simulink library "foc_blocks"  (R2020b)
settings: Solver=ode45  StartTime=0.0  StopTime=10.0  RelTol=1e-3  EnableMultiTasking=on
values from neighbouring files (symbols this model uses):
  ClockFrequency = 100    [setup_DF_fixp16_alu_av.m]    (also in setup_sim_DF_fixp16_alu.m; setup_verify_DF_fixp16_alu.m)
  constfractionlengthIn = 10    [setup_DF_fixp16_alu_av.m]    (also in setup_sim_DF_fixp16_alu.m; setup_verify_DF_fixp16_alu.m)
  constwordlengthIn = 16    [setup_DF_fixp16_alu_av.m]    (also in setup_sim_DF_fixp16_alu.m; setup_verify_DF_fixp16_alu.m)
  DSPBASampleTime = FoldingFactor / (ClockFrequency * 1e6)    (= 5e-06)    [setup_DF_fixp16_alu_av.m]    (also in setup_sim_DF_fixp16_alu.m; setup_verify_DF_fixp16_alu.m)
  FoldingFactor = 500    [setup_DF_fixp16_alu_av.m]    (also in setup_sim_DF_fixp16_alu.m; setup_verify_DF_fixp16_alu.m)
undefined symbols (not defined in the file or in its folder): AdvDSPBChannelOutDisplay, dpoly, dspba_ChannelInVis, dspba_ChannelOutVis, dspba_internal_get_channel_ports, evalAionMaskParam, latency, primtype, value, x
libraries: DSPBAPrim x559, AlteraGenericMotorLibrary x20, $bdroot x9, DSPBAUtilities x4, DSPBAControl x4
(part 1 of 6)
settings Model: Creator=tchau  LastModifiedBy=shiyaowa
settings DataIOCC: LimitDataPoints=on  SaveFormat=Array  ReturnWorkspaceOutputs=off
settings OptimizationCC: LifeSpan=inf
settings DebuggingCC: SolverPrmCheckMsg=warning  SFUnexpectedBacktrackingDiag=warning  SFNoUnconditionalDefaultTransitionDiag=warning  SFExecutionAtInitializationDiag=none  ArithmeticOperatorsInVariantConditions=warning
settings HardwareCC: ProdBitPerPointer=32  ProdBitPerSizeT=32  ProdBitPerPtrDiffT=32  ProdLargestAtomicFloat=None  ProdIntDivRoundTo=Undefined  ProdEndianess=Unspecified  ProdWordSize=32  ProdHWDeviceType=32-bit Generic
settings ModelReferenceCC: PropagateSignalLabelsOutOfModel=off
settings SFSimCC: SimUseLocalCustomCode=off  CustomCodeUndefinedFunction=UseInterfaceOnly
settings RTWCC: RTWUseLocalCustomCode=off
settings CodeAppCC: StateflowObjectComments=on
settings GRTTargetCC: TargetLangStandard=C89/C90 (ANSI)
settings ConfigComp: CovMetricSettings=dw  CovSaveCumulativeToWorkspaceVar=on  CovSaveSingleToWorkspaceVar=on  CovExternalEMLEnable=off

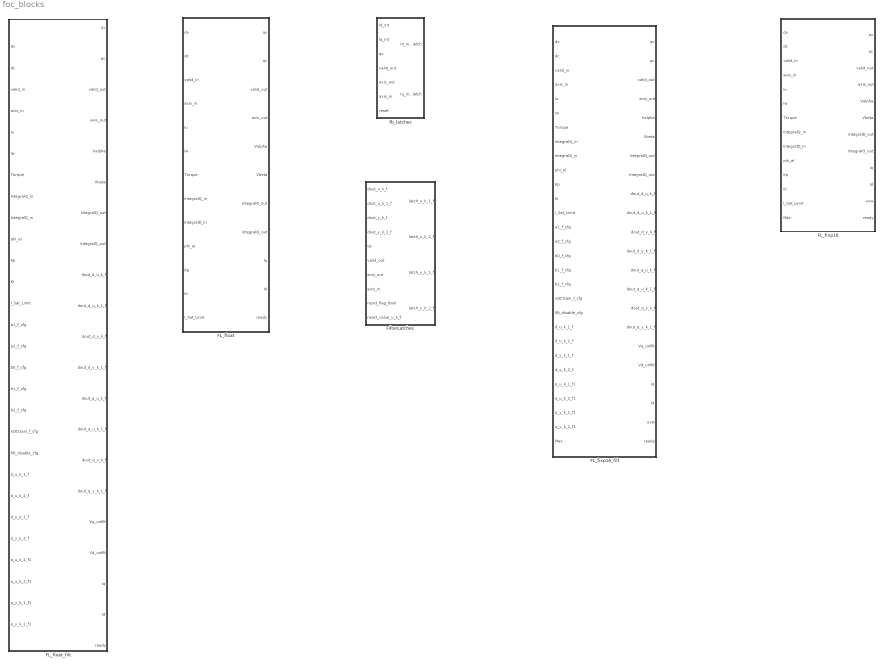
== system foc_blocks ==
  FL_fixp16 : Subsystem
  FL_fixp16_filt : Subsystem
  FL_float : Subsystem
  FL_float_filt : Subsystem
  FilterLatches : Subsystem
  fb_latches : Subsystem

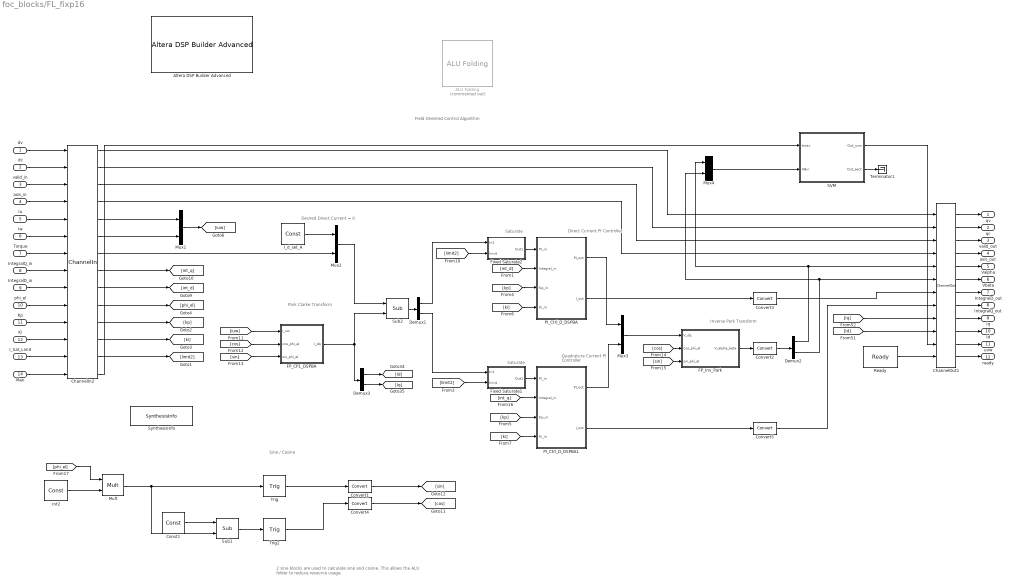
== system foc_blocks/FL_fixp16 ==
  note: Field Oriented Control Algorithm
  note: Sine / Cosine
  note: Saturate
  note: Saturate
  note: Park Clarke
      |  Transform
  note: Inverse Park
      |  Transform
  note: Desired Direct Current = 0
  note: Direct Current
      | PI Controller
  note: Quadrature Current
      | PI Controller
  note: 2 sine blocks are used to calculate sine and cosine.
      | This allows the ALU folder to reduce resource usage.
  dv : Inport
  dc : Inport  Port=2
  valid_in : Inport  Port=3
  axis_in : Inport  Port=4
  Iu : Inport  Port=5
  Iw : Inport  Port=6
  Torque : Inport  Port=7
  IntegralQ_in : Inport  Port=8
  IntegralD_in : Inport  Port=9
  phi_el : Inport  Port=10
  Kp : Inport  Port=11
  Ki : Inport  Port=12
  I_Sat_Limit : Inport  Port=13
  Max : Inport  Port=14
  ALU Folding : DSPBAUtilities/ALU Folding  Description=Enables the new folder. When this block is placed in a subsystem, all primitive subsystems at the level it is placed and below will be passed to the folder. DSP Builder will then generate folded subsystems which can be placed back into the existing design.  Commented=on  version=20130913  genModelFileName=folded_model.xml  sampleRate=SampleRate  numChannels=1  maxLatency=LatencyConstraint  inputFormat=Parallel  outputFormat=Parallel  latchOutputs=off  originalRate=off  hasIdleState=off  padInputs=off  simRate=Data rate
  Altera DSP Builder Advanced : AlteraGenericMotorLibrary/FP_Cur_Ctrl_DSPBA/Altera DSP Builder Advanced  SystemSampleTime=-1  VariantActivationTime=update diagram  Latency=0  AutoFrameSizeCalculation=off
  ChannelIn2 : DSPBAPrim/ChannelIn  primtype=channelin  nInputs=dspba_internal_get_channel_ports(gcb)  nOutputs=dspba_internal_get_channel_ports(gcb)  omode=Inherit via internal rule  otype=sfix(16)  scale=2^-15  rndmethod=Unbiased  factor=1  satmethod=Symmetric  shift_vec=[0 1 2 -1]  value=12  inPortNames=['v'; 'c'; '0'; '1'; '2'; '3'; '4'; '5'; '6'; '7'; '8'; '9'; 'A'; 'B'; 'D'; 'E'; 'F'; 'G'; 'H'; 'I'; 'J'; 'K'; 'L'; 'M'; 'N'; 'O'; 'P'; 'Q'; 'R'; 'S'; 'T'; 'U'; 'W'; 'X'; 'Y'; 'Z']  outPortNames=['v'; 'c'; '0'; '1'; '2'; '3'; '4'; '5'; '6'; '7'; '8'; '9'; 'A'; 'B'; 'D'; 'E'; 'F'; 'G'; 'H'; 'I'; 'J'; 'K'; 'L'; 'M'; 'N'; 'O'; 'P'; 'Q'; 'R'; 'S'; 'T'; 'U'; 'W'; 'X'; 'Y'; 'Z']  dspbaimage=dspba_prim.jpg  text=fprintf('In');  style=Optimised  dataSignals=12  foldingEnabled=off  channels=1  sampleRate=200  packetBeginPresent=off  packetBeginEnabled=off  visibilities=dspba_ChannelInVis(gcb)  latencyCorrection=0  scheduleOrigin=off  version=20141013
  ChannelOut1 : DSPBAPrim/ChannelOut  primtype=channelout  nInputs=dspba_internal_get_channel_ports(gcb)  nOutputs=dspba_internal_get_channel_ports(gcb)  omode=Inherit via internal rule  otype=sfix(16)  scale=2^-15  rndmethod=Unbiased  factor=1  satmethod=Symmetric  shift_vec=[0 1 2 -1]  value=10  inPortNames=['v'; 'c'; '0'; '1'; '2'; '3'; '4'; '5'; '6'; '7'; '8'; '9'; 'A'; 'B'; 'D'; 'E'; 'F'; 'G'; 'H'; 'I'; 'J'; 'K'; 'L'; 'M'; 'N'; 'O'; 'P'; 'Q'; 'R'; 'S'; 'T'; 'U'; 'W'; 'X'; 'Y'; 'Z']  outPortNames=['v'; 'c'; '0'; '1'; '2'; '3'; '4'; '5'; '6'; '7'; '8'; '9'; 'A'; 'B'; 'D'; 'E'; 'F'; 'G'; 'H'; 'I'; 'J'; 'K'; 'L'; 'M'; 'N'; 'O'; 'P'; 'Q'; 'R'; 'S'; 'T'; 'U'; 'W'; 'X'; 'Y'; 'Z']  dspbaimage=dspba_prim.jpg  text=fprintf('Out%s', AdvDSPBChannelOutDisplay(latency));  style=Optimised  dataSignals=10  foldingEnabled=off  channels=1  sampleRate=200  packetBeginPresent=off  packetBeginEnabled=off  visibilities=dspba_ChannelOutVis(gcb)  latency=22  latencyCorrection=0  version=20141013
  Const1 : DSPBAPrim/Const  primtype=const  nInputs=0  nOutputs=1  omode=Specify via dialog  otype=constOTypeIn  scale=constScaleIn  rndmethod=Unbiased  factor=1  satmethod=Symmetric  shift_vec=[0 1 2 -1]  value=1/2  inPortNames=['+'; '+';]  outPortNames=[' ']  dspbaimage=dspba_prim.jpg  text=fprintf('%s', num2str(value));  style=Optimised  visibilities=8 + 1024  floatPrecision=float26_m17  version=20120820
  Convert{1,3..5} (4 alike) : DSPBAPrim/Convert  primtype=convert  nInputs=1  nOutputs=1  omode=Specify via dialog  otype=constOTypeIn  scale=constScaleIn  rndmethod=Truncate  factor=1  satmethod=None  shift_vec=[0 1 2 -1]  value=round([0:255]/17)  inPortNames=[' '; ' ';]  outPortNames=[' '; 'c']  dspbaimage=dspba_prim.jpg  text=fprintf('convert');  style=Optimised  visibilities=8+64+256  clipdetect=off  floatPrecision=float32_m23  advOptions=[]  version=20130211
  Convert2 : DSPBAPrim/Convert  primtype=convert  nInputs=1  nOutputs=1  omode=Specify via dialog  otype=constOType  scale=constScale  rndmethod=Truncate  factor=1  satmethod=None  shift_vec=[0 1 2 -1]  value=round([0:255]/17)  inPortNames=[' '; ' ';]  outPortNames=[' '; 'c']  dspbaimage=dspba_prim.jpg  text=fprintf('convert');  style=Optimised  visibilities=8+64+256  clipdetect=off  floatPrecision=float32_m23  advOptions=[]  version=20130211
  Demux1 : Demux  Outputs=2
  Demux2 : Demux  Outputs=2
  Demux3 : Demux  Outputs=2
  FP_CP1_DSPBA : Subsystem  Description=Clarke & Park Transforms
      mask Display: color('white');port_label('output', 1, 'I_dq'); port_label('input', 1, 'I_uw');port_label('input', 2, 'cos_phi');port_label('input', 3, 'sin_phi');
  FP_Inv_Park : Subsystem  Description=Inverse Park & Clarke transforms
      mask Display: color('white');port_label('output', 1, 'V_alpha_beta'); port_label('input', 1, 'V_dq');port_label('input', 2, 'cos_phi');port_label('input', 3, 'sin_phi');
  Fixed Saturate1 : Subsystem
  Fixed Saturate2 : Subsystem
  I_d_set_A : DSPBAPrim/Const  primtype=const  nInputs=0  nOutputs=1  omode=Specify via dialog  otype=constOTypeIn  scale=constScaleIn  rndmethod=Unbiased  factor=1  satmethod=Symmetric  shift_vec=[0 1 2 -1]  value=0  inPortNames=['+'; '+';]  outPortNames=[' ']  dspbaimage=dspba_prim.jpg  text=fprintf('%s', num2str(value));  style=Optimised  visibilities=8 + 1024  floatPrecision=float32_m23  version=20120820
  Mult : DSPBAPrim/Mult  primtype=mult  nInputs=2  nOutputs=1  omode=Specify via dialog  otype=constOTypeIn  scale=constScaleIn  rndmethod=Unbiased  factor=1  satmethod=Symmetric  shift_vec=[0 1 2 -1]  value=0  inPortNames=[' '; ' ';]  outPortNames=[' ']  dspbaimage=dspba_prim.jpg  text=fprintf('X');  style=Optimised  visibilities=8  floatPrecision=float32_m23  floatRounding=correct  advOptions=[]  version=20130115
  Mux{1..4} (4 alike) : Mux  Inputs=2
  PI_Ctrl_D_DSPBA : Subsystem
  PI_Ctrl_D_DSPBA1 : Subsystem
  Ready : DSPBAPrim/Ready  primtype=ready  nInputs=0  nOutputs=1  omode=Inherit via internal rule  otype=ufix(1)  scale=2^-0  rndmethod=Unbiased  factor=1  satmethod=Asymmetric  shift_vec=[]  value=1  inPortNames=['']  outPortNames=[' ']  dspbaimage=dspba_prim.jpg  text=fprintf('Ready');  style=Processor  visibilities=0  floatPrecision=float32_m23  version=20131024
  SVM : Subsystem
  Sub1 : DSPBAPrim/Sub  primtype=sub  nInputs=2  nOutputs=1  omode=Inherit via internal rule  otype=sfix(16)  scale=2^-15  rndmethod=Unbiased  factor=1  satmethod=Symmetric  shift_vec=[0 1 2 -1]  value=0  inPortNames=['+'; '-';]  outPortNames=[' ']  dspbaimage=dspba_prim.jpg  text=fprintf('-');  style=Optimised  visibilities=8  floatRounding=correct  advOptions=[]  version=20130115
  Sub2 : DSPBAPrim/Sub  primtype=sub  nInputs=2  nOutputs=1  omode=Inherit via internal rule  otype=sfix(16)  scale=2^-15  rndmethod=Unbiased  factor=1  satmethod=Symmetric  shift_vec=[0 1 2 -1]  value=0  inPortNames=['+'; '-';]  outPortNames=[' ']  dspbaimage=dspba_prim.jpg  text=fprintf('-');  style=Optimised  visibilities=8  floatRounding=correct  advOptions=[]  version=20130115
  SynthesisInfo : DSPBAPrim/SynthesisInfo  primtype=synthinfo  nInputs=0  nOutputs=0  omode=Inherit via internal rule  otype=sfix(16)  scale=2^-15  rndmethod=Truncate  factor=1  satmethod=Symmetric  shift_vec=[0 1 2 -1]  value=99  inPortNames=[' '; ' ';]  outPortNames=[' ']  dspbaimage=dspba_prim_ctrl.jpg  text=fprintf('Style=%s', style);  style=Scheduled  visibilities=32768  constraintInUse=off  constraintRelation=>  constraintLimit=2  bitAccurate=off  version=20150220
  Terminator1 : Terminator
  Trig : DSPBAPrim/Trig  primtype=trigfunc  nInputs=1  nOutputs=1  omode=Inherit via internal rule  otype=sfix(16)  scale=2^-15  rndmethod=Unbiased  factor=1  satmethod=Symmetric  shift_vec=[0 1 2 -1]  value=round([0:255]/17)  inPortNames=[' '; ' ';]  outPortNames=[' ']  dspbaimage=dspba_prim_float.jpg  text=fprintf('sin(a)');  style=Optimised  visibilities=2^17+2^18  functionExpr=sin(pi*x)  advOptions=[]  version=20140803
  Trig2 : DSPBAPrim/Trig  primtype=trigfunc  nInputs=1  nOutputs=1  omode=Inherit via internal rule  otype=sfix(16)  scale=2^-15  rndmethod=Unbiased  factor=1  satmethod=Symmetric  shift_vec=[0 1 2 -1]  value=round([0:255]/17)  inPortNames=[' '; ' ';]  outPortNames=[' ']  dspbaimage=dspba_prim_float.jpg  text=fprintf('sin(a)');  style=Optimised  visibilities=2^17+2^18  functionExpr=sin(pi*x)  advOptions=[]  version=20140803
  cst2 : DSPBAPrim/Const  primtype=const  nInputs=0  nOutputs=1  omode=Specify via dialog  otype=constOTypeIn  scale=constScaleIn  rndmethod=Unbiased  factor=1  satmethod=Symmetric  shift_vec=[0 1 2 -1]  value=2  inPortNames=['+'; '+';]  outPortNames=[' ']  dspbaimage=dspba_prim.jpg  text=fprintf('%s', num2str(value));  style=Optimised  visibilities=8 + 1024  floatPrecision=float26_m17  version=20120820
  qv : Outport
  qc : Outport  Port=2
  valid_out : Outport  Port=3
  axis_out : Outport  Port=4
  Valpha : Outport  Port=5
  Vbeta : Outport  Port=6
  IntegralD_out : Outport  Port=7
  IntegralQ_out : Outport  Port=8
  Iq : Outport  Port=9
  Id : Outport  Port=10
  uvw : Outport  Port=11
  ready : Outport  Port=12
  wires:
  SVM/2(Out_sect) -> Terminator1/1
  Ready/1 -> ChannelOut1/12
  ChannelOut1/12 -> ready/1
  SVM/1(Out_uvw) -> ChannelOut1/11
  ChannelOut1/11 -> uvw/1
  ChannelIn2/14 -> SVM/1(tmax)
  Max/1 -> ChannelIn2/14
  Mux4/1 -> SVM/2(ABin)
  Mux2/1 -> Sub2/1
  ChannelIn2/12 -> [ki]
  ChannelIn2/11 -> [kp]
  ChannelIn2/10 -> [phi_el]
  ChannelIn2/9 -> [int_d]
  ChannelIn2/8 -> [int_q]
  ChannelIn2/7 -> Mux2/2
  ChannelIn2/6 -> Mux1/2
  ChannelIn2/5 -> Mux1/1
  Sub1/1 -> Trig2/1
  Mult/1 -> Sub1/2, Trig/1
  Const1/1 -> Sub1/1
  Convert4/1 -> [cos]
  Convert1/1 -> [sin]
  Trig2/1 -> Convert4/1
  Trig/1 -> Convert1/1
  cst2/1 -> Mult/2
  [phi_el] -> Mult/1
  ChannelIn2/4 -> ChannelOut1/4
  [sin] -> FP_Inv_Park/3(sin_phi_el)
  [cos] -> FP_Inv_Park/2(cos_phi_el)
  Convert2/1 -> Demux2/1
  Mux1/1 -> [iuw]
  [sin] -> FP_CP1_DSPBA/3(sin_phi_el)
  [cos] -> FP_CP1_DSPBA/2(cos_phi_el)
  [iuw] -> FP_CP1_DSPBA/1(I_uw)
  [limit2] -> Fixed Saturate2/2(limit)
  [ki] -> PI_Ctrl_D_DSPBA/4(Ki_in)
  [kp] -> PI_Ctrl_D_DSPBA/3(Kp_in)
  [int_d] -> PI_Ctrl_D_DSPBA/2(Integral_in)
  [limit2] -> Fixed Saturate1/2(limit)
  [ki] -> PI_Ctrl_D_DSPBA1/4(Ki_in)
  [kp] -> PI_Ctrl_D_DSPBA1/3(Kp_in)
  [int_q] -> PI_Ctrl_D_DSPBA1/2(Integral_in)
  Demux1/2 -> Fixed Saturate1/1(In1)
  Demux1/1 -> Fixed Saturate2/1(In1)
  Sub2/1 -> Demux1/1
  I_d_set_A/1 -> Mux2/1
  Demux2/2 -> ChannelOut1/6, Mux4/2
  Demux2/1 -> ChannelOut1/5, Mux4/1
  FP_Inv_Park/1(V_alpha_beta) -> Convert2/1
  Mux3/1 -> FP_Inv_Park/1(V_dq)
  PI_Ctrl_D_DSPBA1/1(PI_out) -> Mux3/2
  PI_Ctrl_D_DSPBA/1(PI_out) -> Mux3/1
  Convert3/1 -> ChannelOut1/7
  PI_Ctrl_D_DSPBA/2(I_out) -> Convert3/1
  Convert5/1 -> ChannelOut1/8
  PI_Ctrl_D_DSPBA1/2(I_out) -> Convert5/1
  Fixed Saturate2/1(Out1) -> PI_Ctrl_D_DSPBA/1(PI_in)
  Fixed Saturate1/1(Out1) -> PI_Ctrl_D_DSPBA1/1(PI_in)
  ChannelIn2/3 -> ChannelOut1/3
  ChannelIn2/2 -> ChannelOut1/2
  ChannelIn2/1 -> ChannelOut1/1
  dv/1 -> ChannelIn2/1
  dc/1 -> ChannelIn2/2
  valid_in/1 -> ChannelIn2/3
  axis_in/1 -> ChannelIn2/4
  Iu/1 -> ChannelIn2/5
  Iw/1 -> ChannelIn2/6
  Torque/1 -> ChannelIn2/7
  IntegralQ_in/1 -> ChannelIn2/8
  IntegralD_in/1 -> ChannelIn2/9
  phi_el/1 -> ChannelIn2/10
  Kp/1 -> ChannelIn2/11
  Ki/1 -> ChannelIn2/12
  ChannelOut1/1 -> qv/1
  ChannelOut1/2 -> qc/1
  ChannelOut1/3 -> valid_out/1
  ChannelOut1/4 -> axis_out/1
  ChannelOut1/5 -> Valpha/1
  ChannelOut1/6 -> Vbeta/1
  ChannelOut1/7 -> IntegralD_out/1
  ChannelOut1/8 -> IntegralQ_out/1
  FP_CP1_DSPBA/1(I_dq) -> Sub2/2, Demux3/1
  Demux3/1 -> [Id]
  Demux3/2 -> [Iq]
  [Iq] -> ChannelOut1/9
  [Id] -> ChannelOut1/10
  ChannelOut1/9 -> Iq/1
  ChannelOut1/10 -> Id/1
  I_Sat_Limit/1 -> ChannelIn2/13
  ChannelIn2/13 -> [limit2]

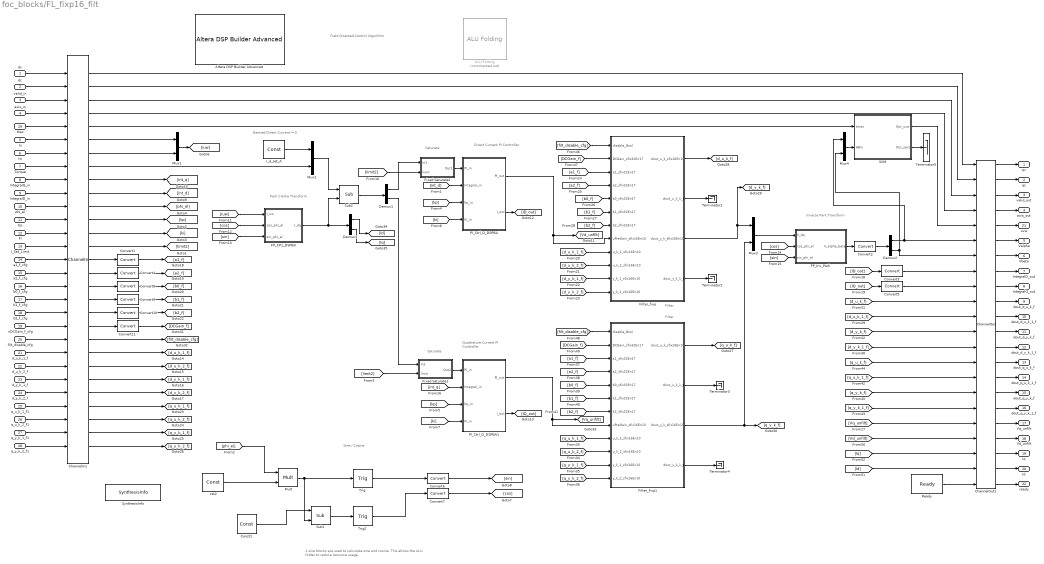
== system foc_blocks/FL_fixp16_filt ==
  note: Sine / Cosine
  note: Filter
  note: Filter
  note: Field Oriented Control Algorithm
  note: Saturate
  note: Saturate
  note: Park Clarke
      |  Transform
  note: Inverse Park
      |  Transform
  note: Desired Direct Current = 0
  note: Direct Current
      | PI Controller
  note: Quadrature Current
      | PI Controller
  note: 2 sine blocks are used to calculate sine and cosine.
      | This allows the ALU folder to reduce resource usage.
  dv : Inport
  dc : Inport  Port=2
  valid_in : Inport  Port=3
  axis_in : Inport  Port=4
  Iu : Inport  Port=5
  Iw : Inport  Port=6
  Torque : Inport  Port=7
  IntegralQ_in : Inport  Port=8
  IntegralD_in : Inport  Port=9
  phi_el : Inport  Port=10
  Kp : Inport  Port=11
  Ki : Inport  Port=12
  I_Sat_Limit : Inport  Port=13
  a1_f_cfg : Inport  Port=14
  a2_f_cfg : Inport  Port=15
  b0_f_cfg : Inport  Port=16
  b1_f_cfg : Inport  Port=17
  b2_f_cfg : Inport  Port=18
  xDCGain_f_cfg : Inport  Port=19
  filt_disable_cfg : Inport  Port=20
  d_u_k_1_f : Inport  Port=21
  d_u_k_2_f : Inport  Port=22
  d_y_k_1_f : Inport  Port=23
  d_y_k_2_f : Inport  Port=24
  q_u_k_1_f1 : Inport  Port=25
  q_u_k_2_f1 : Inport  Port=26
  q_y_k_1_f1 : Inport  Port=27
  q_y_k_2_f1 : Inport  Port=28
  Max : Inport  Port=29
  ALU Folding : DSPBAUtilities/ALU Folding  Description=Enables the new folder. When this block is placed in a subsystem, all primitive subsystems at the level it is placed and below will be passed to the folder. DSP Builder will then generate folded subsystems which can be placed back into the existing design.  Commented=on  version=20130913  genModelFileName=folded_model.xml  sampleRate=SampleRate  numChannels=1  maxLatency=LatencyConstraint  inputFormat=Parallel  outputFormat=Parallel  latchOutputs=off  originalRate=off  hasIdleState=off  padInputs=off  simRate=Data rate
  Altera DSP Builder Advanced : AlteraGenericMotorLibrary/FP_Cur_Ctrl_DSPBA/Altera DSP Builder Advanced  SystemSampleTime=-1  VariantActivationTime=update diagram  Latency=0  AutoFrameSizeCalculation=off
  ChannelIn1 : DSPBAPrim/ChannelIn  primtype=channelin  nInputs=dspba_internal_get_channel_ports(gcb)  nOutputs=dspba_internal_get_channel_ports(gcb)  omode=Inherit via internal rule  otype=sfix(16)  scale=2^-15  rndmethod=Unbiased  factor=1  satmethod=Symmetric  shift_vec=[0 1 2 -1]  value=27  inPortNames=['v'; 'c'; '0'; '1'; '2'; '3'; '4'; '5'; '6'; '7'; '8'; '9'; 'A'; 'B'; 'D'; 'E'; 'F'; 'G'; 'H'; 'I'; 'J'; 'K'; 'L'; 'M'; 'N'; 'O'; 'P'; 'Q'; 'R'; 'S'; 'T'; 'U'; 'W'; 'X'; 'Y'; 'Z']  outPortNames=['v'; 'c'; '0'; '1'; '2'; '3'; '4'; '5'; '6'; '7'; '8'; '9'; 'A'; 'B'; 'D'; 'E'; 'F'; 'G'; 'H'; 'I'; 'J'; 'K'; 'L'; 'M'; 'N'; 'O'; 'P'; 'Q'; 'R'; 'S'; 'T'; 'U'; 'W'; 'X'; 'Y'; 'Z']  dspbaimage=dspba_prim.jpg  text=fprintf('In');  style=Optimised  dataSignals=27  foldingEnabled=off  channels=1  sampleRate=ClockFrequency/FoldingFactor  packetBeginPresent=off  packetBeginEnabled=off  visibilities=dspba_ChannelInVis(gcb)  latencyCorrection=0  scheduleOrigin=off  version=20141013
  ChannelOut1 : DSPBAPrim/ChannelOut  primtype=channelout  nInputs=dspba_internal_get_channel_ports(gcb)  nOutputs=dspba_internal_get_channel_ports(gcb)  omode=Inherit via internal rule  otype=sfix(16)  scale=2^-15  rndmethod=Unbiased  factor=1  satmethod=Symmetric  shift_vec=[0 1 2 -1]  value=20  inPortNames=['v'; 'c'; '0'; '1'; '2'; '3'; '4'; '5'; '6'; '7'; '8'; '9'; 'A'; 'B'; 'D'; 'E'; 'F'; 'G'; 'H'; 'I'; 'J'; 'K'; 'L'; 'M'; 'N'; 'O'; 'P'; 'Q'; 'R'; 'S'; 'T'; 'U'; 'W'; 'X'; 'Y'; 'Z']  outPortNames=['v'; 'c'; '0'; '1'; '2'; '3'; '4'; '5'; '6'; '7'; '8'; '9'; 'A'; 'B'; 'D'; 'E'; 'F'; 'G'; 'H'; 'I'; 'J'; 'K'; 'L'; 'M'; 'N'; 'O'; 'P'; 'Q'; 'R'; 'S'; 'T'; 'U'; 'W'; 'X'; 'Y'; 'Z']  dspbaimage=dspba_prim.jpg  text=fprintf('Out%s', AdvDSPBChannelOutDisplay(latency));  style=Optimised  dataSignals=20  foldingEnabled=off  channels=1  sampleRate=ClockFrequency/FoldingFactor  packetBeginPresent=off  packetBeginEnabled=off  visibilities=dspba_ChannelOutVis(gcb)  latency=17  latencyCorrection=0  version=20141013
  Const1 : DSPBAPrim/Const  primtype=const  nInputs=0  nOutputs=1  omode=Specify via dialog  otype=constOTypeIn  scale=constScaleIn  rndmethod=Unbiased  factor=1  satmethod=Symmetric  shift_vec=[0 1 2 -1]  value=1/2  inPortNames=['+'; '+';]  outPortNames=[' ']  dspbaimage=dspba_prim.jpg  text=fprintf('%s', num2str(value));  style=Optimised  visibilities=8 + 1024  floatPrecision=float26_m17  version=20120820
  Convert{1,3..11} (10 alike) : DSPBAPrim/Convert  primtype=convert  nInputs=1  nOutputs=1  omode=Specify via dialog  otype=constOTypeIn  scale=constScaleIn  rndmethod=Truncate  factor=1  satmethod=None  shift_vec=[0 1 2 -1]  value=round([0:255]/17)  inPortNames=[' '; ' ';]  outPortNames=[' '; 'c']  dspbaimage=dspba_prim.jpg  text=fprintf('convert');  style=Optimised  visibilities=8+64+256  clipdetect=off  floatPrecision=float32_m23  advOptions=[]  version=20130211
  Convert2 : DSPBAPrim/Convert  primtype=convert  nInputs=1  nOutputs=1  omode=Specify via dialog  otype=constOType  scale=constScale  rndmethod=Truncate  factor=1  satmethod=None  shift_vec=[0 1 2 -1]  value=round([0:255]/17)  inPortNames=[' '; ' ';]  outPortNames=[' '; 'c']  dspbaimage=dspba_prim.jpg  text=fprintf('convert');  style=Optimised  visibilities=8+64+256  clipdetect=off  floatPrecision=float32_m23  advOptions=[]  version=20130211
  Demux1 : Demux  Outputs=2
  Demux2 : Demux  Outputs=2
  Demux3 : Demux  Outputs=2
  FP_CP1_DSPBA : Subsystem  Description=Clarke & Park Transforms
      mask Display: color('white');port_label('output', 1, 'I_dq'); port_label('input', 1, 'I_uw');port_label('input', 2, 'cos_phi');port_label('input', 3, 'sin_phi');
  FP_Inv_Park : Subsystem  Description=Inverse Park & Clarke transforms
      mask Display: color('white');port_label('output', 1, 'V_alpha_beta'); port_label('input', 1, 'V_dq');port_label('input', 2, 'cos_phi');port_label('input', 3, 'sin_phi');
  Filter_fixp : Subsystem
  Filter_fixp1 : Subsystem
  Fixed Saturate1 : Subsystem
  Fixed Saturate2 : Subsystem
  I_d_set_A : DSPBAPrim/Const  primtype=const  nInputs=0  nOutputs=1  omode=Specify via dialog  otype=constOTypeIn  scale=constScaleIn  rndmethod=Unbiased  factor=1  satmethod=Symmetric  shift_vec=[0 1 2 -1]  value=0  inPortNames=['+'; '+';]  outPortNames=[' ']  dspbaimage=dspba_prim.jpg  text=fprintf('%s', num2str(value));  style=Optimised  visibilities=8 + 1024  floatPrecision=float32_m23  version=20120820
  Mult : DSPBAPrim/Mult  primtype=mult  nInputs=2  nOutputs=1  omode=Specify via dialog  otype=constOTypeIn  scale=constScaleIn  rndmethod=Unbiased  factor=1  satmethod=Symmetric  shift_vec=[0 1 2 -1]  value=0  inPortNames=[' '; ' ';]  outPortNames=[' ']  dspbaimage=dspba_prim.jpg  text=fprintf('X');  style=Optimised  visibilities=8  floatPrecision=float32_m23  floatRounding=correct  advOptions=[]  version=20130115
  Mux{1..4} (4 alike) : Mux  Inputs=2
  PI_Ctrl_D_DSPBA : Subsystem
  PI_Ctrl_D_DSPBA1 : Subsystem
  Ready : DSPBAPrim/Ready  primtype=ready  nInputs=0  nOutputs=1  omode=Inherit via internal rule  otype=ufix(1)  scale=2^-0  rndmethod=Unbiased  factor=1  satmethod=Asymmetric  shift_vec=[]  value=1  inPortNames=['']  outPortNames=[' ']  dspbaimage=dspba_prim.jpg  text=fprintf('Ready');  style=Processor  visibilities=0  floatPrecision=float32_m23  version=20131024
  SVM : Subsystem
  Sub1 : DSPBAPrim/Sub  primtype=sub  nInputs=2  nOutputs=1  omode=Inherit via internal rule  otype=sfix(16)  scale=2^-15  rndmethod=Unbiased  factor=1  satmethod=Symmetric  shift_vec=[0 1 2 -1]  value=0  inPortNames=['+'; '-';]  outPortNames=[' ']  dspbaimage=dspba_prim.jpg  text=fprintf('-');  style=Optimised  visibilities=8  floatRounding=correct  advOptions=[]  version=20130115
  Sub2 : DSPBAPrim/Sub  primtype=sub  nInputs=2  nOutputs=1  omode=Inherit via internal rule  otype=sfix(16)  scale=2^-15  rndmethod=Unbiased  factor=1  satmethod=Symmetric  shift_vec=[0 1 2 -1]  value=0  inPortNames=['+'; '-';]  outPortNames=[' ']  dspbaimage=dspba_prim.jpg  text=fprintf('-');  style=Optimised  visibilities=8  floatRounding=correct  advOptions=[]  version=20130115
  SynthesisInfo : DSPBAPrim/SynthesisInfo  primtype=synthinfo  nInputs=0  nOutputs=0  omode=Inherit via internal rule  otype=sfix(16)  scale=2^-15  rndmethod=Truncate  factor=1  satmethod=Symmetric  shift_vec=[0 1 2 -1]  value=99  inPortNames=[' '; ' ';]  outPortNames=[' ']  dspbaimage=dspba_prim_ctrl.jpg  text=fprintf('Style=%s', style);  style=Scheduled  visibilities=32768  constraintInUse=off  constraintRelation=>  constraintLimit=2  bitAccurate=off  version=20150220
  Terminator{1..5} (5 alike) : Terminator
  Trig : DSPBAPrim/Trig  primtype=trigfunc  nInputs=1  nOutputs=1  omode=Inherit via internal rule  otype=sfix(16)  scale=2^-15  rndmethod=Unbiased  factor=1  satmethod=Symmetric  shift_vec=[0 1 2 -1]  value=round([0:255]/17)  inPortNames=[' '; ' ';]  outPortNames=[' ']  dspbaimage=dspba_prim_float.jpg  text=fprintf('sin(a)');  style=Optimised  visibilities=2^17+2^18  functionExpr=sin(pi*x)  advOptions=[]  version=20140803
  Trig2 : DSPBAPrim/Trig  primtype=trigfunc  nInputs=1  nOutputs=1  omode=Inherit via internal rule  otype=sfix(16)  scale=2^-15  rndmethod=Unbiased  factor=1  satmethod=Symmetric  shift_vec=[0 1 2 -1]  value=round([0:255]/17)  inPortNames=[' '; ' ';]  outPortNames=[' ']  dspbaimage=dspba_prim_float.jpg  text=fprintf('sin(a)');  style=Optimised  visibilities=2^17+2^18  functionExpr=sin(pi*x)  advOptions=[]  version=20140803
  cst2 : DSPBAPrim/Const  primtype=const  nInputs=0  nOutputs=1  omode=Specify via dialog  otype=constOTypeIn  scale=constScaleIn  rndmethod=Unbiased  factor=1  satmethod=Symmetric  shift_vec=[0 1 2 -1]  value=2  inPortNames=['+'; '+';]  outPortNames=[' ']  dspbaimage=dspba_prim.jpg  text=fprintf('%s', num2str(value));  style=Optimised  visibilities=8 + 1024  floatPrecision=float26_m17  version=20120820
  qv : Outport
  qc : Outport  Port=2
  valid_out : Outport  Port=3
  axis_out : Outport  Port=4
  Valpha : Outport  Port=5
  Vbeta : Outport  Port=6
  IntegralD_out : Outport  Port=7
  IntegralQ_out : Outport  Port=8
  dout_d_u_k_f : Outport  Port=9
  dout_d_u_k_1_f : Outport  Port=10
  dout_d_y_k_f : Outport  Port=11
  dout_d_y_k_1_f : Outport  Port=12
  dout_q_u_k_f : Outport  Port=13
  dout_q_u_k_1_f : Outport  Port=14
  dout_q_y_k_f : Outport  Port=15
  dout_q_y_k_1_f : Outport  Port=16
  Vq_unfilt : Outport  Port=17
  Vd_unfilt : Outport  Port=18
  Iq : Outport  Port=19
  Id : Outport  Port=20
  uvw : Outport  Port=21
  ready : Outport  Port=22
  wires:
  Sub1/1 -> Trig2/1
  Mult/1 -> Sub1/2, Trig/1
  Const1/1 -> Sub1/1
  Convert7/1 -> [cos]
  Convert6/1 -> [sin]
  Trig2/1 -> Convert7/1
  Trig/1 -> Convert6/1
  cst2/1 -> Mult/2
  [phi_el] -> Mult/1
  PI_Ctrl_D_DSPBA1/1(PI_out) -> Filter_fixp1/8(uPreGain_sfix16En10), [Vq_unfilt]
  PI_Ctrl_D_DSPBA/1(PI_out) -> [Vd_unfilt], Filter_fixp/8(uPreGain_sfix16En10)
  Demux3/2 -> [Iq]
  Demux3/1 -> [Id]
  [DCGain_f] -> Filter_fixp1/2(DCGain_sfix32En17)
  [filt_disable_cfg] -> Filter_fixp1/1(disable_Bool)
  Filter_fixp1/1(dout_u_k_sfix16En10) -> [q_u_k_f]
  Filter_fixp1/2(dout_u_k_1_f) -> Terminator3/1
  Filter_fixp1/4(dout_y_k_1_f) -> Terminator4/1
  [a1_f] -> Filter_fixp1/3(a1_sfix32En17)
  [a2_f] -> Filter_fixp1/4(a2_sfix32En17)
  [b0_f] -> Filter_fixp1/5(b0_sfix32En17)
  [b1_f] -> Filter_fixp1/6(b1_sfix32En17)
  [b2_f] -> Filter_fixp1/7(b2_sfix32En17)
  [q_y_k_2_f] -> Filter_fixp1/12(y_k_2_sfix16En10)
  [q_y_k_1_f] -> Filter_fixp1/11(y_k_1_sfix16En10)
  [q_u_k_2_f] -> Filter_fixp1/10(u_k_2_sfix16En10)
  [q_u_k_1_f] -> Filter_fixp1/9(u_k_1_sfix16En10)
  Filter_fixp1/3(dout_y_k_sfix16En10) -> Mux3/2, [q_y_k_f]
  [DCGain_f] -> Filter_fixp/2(DCGain_sfix32En17)
  [filt_disable_cfg] -> Filter_fixp/1(disable_Bool)
  Filter_fixp/4(dout_y_k_1_f) -> Terminator2/1
  Filter_fixp/2(dout_u_k_1_f) -> Terminator1/1
  Filter_fixp/1(dout_u_k_sfix16En10) -> [d_u_k_f]
  [a1_f] -> Filter_fixp/3(a1_sfix32En17)
  [a2_f] -> Filter_fixp/4(a2_sfix32En17)
  [b0_f] -> Filter_fixp/5(b0_sfix32En17)
  [b1_f] -> Filter_fixp/6(b1_sfix32En17)
  [b2_f] -> Filter_fixp/7(b2_sfix32En17)
  [d_y_k_2_f] -> Filter_fixp/12(y_k_2_sfix16En10)
  [d_y_k_1_f] -> Filter_fixp/11(y_k_1_sfix16En10)
  [d_u_k_2_f] -> Filter_fixp/10(u_k_2_sfix16En10)
  [d_u_k_1_f] -> Filter_fixp/9(u_k_1_sfix16En10)
  Filter_fixp/3(dout_y_k_sfix16En10) -> [d_y_k_f], Mux3/1
  PI_Ctrl_D_DSPBA1/2(I_out) -> [IQ_out]
  PI_Ctrl_D_DSPBA/2(I_out) -> [ID_out]
  ChannelIn1/4 -> ChannelOut1/4
  [sin] -> FP_Inv_Park/3(sin_phi_el)
  [cos] -> FP_Inv_Park/2(cos_phi_el)
  Convert2/1 -> Demux2/1
  [sin] -> FP_CP1_DSPBA/3(sin_phi_el)
  [cos] -> FP_CP1_DSPBA/2(cos_phi_el)
  [iuw] -> FP_CP1_DSPBA/1(I_uw)
  [limit2] -> Fixed Saturate2/2(limit)
  [ki] -> PI_Ctrl_D_DSPBA/4(Ki_in)
  [kp] -> PI_Ctrl_D_DSPBA/3(Kp_in)
  [int_d] -> PI_Ctrl_D_DSPBA/2(Integral_in)
  [limit2] -> Fixed Saturate1/2(limit)
  [ki] -> PI_Ctrl_D_DSPBA1/4(Ki_in)
  [kp] -> PI_Ctrl_D_DSPBA1/3(Kp_in)
  [int_q] -> PI_Ctrl_D_DSPBA1/2(Integral_in)
  Demux1/2 -> Fixed Saturate1/1(In1)
  Demux1/1 -> Fixed Saturate2/1(In1)
  Sub2/1 -> Demux1/1
  Mux2/1 -> Sub2/1
  I_d_set_A/1 -> Mux2/1
  Demux2/2 -> Mux4/2, ChannelOut1/7
  Demux2/1 -> ChannelOut1/6, Mux4/1
  FP_Inv_Park/1(V_alpha_beta) -> Convert2/1
  Mux3/1 -> FP_Inv_Park/1(V_dq)
  Fixed Saturate2/1(Out1) -> PI_Ctrl_D_DSPBA/1(PI_in)
  Fixed Saturate1/1(Out1) -> PI_Ctrl_D_DSPBA1/1(PI_in)
  FP_CP1_DSPBA/1(I_dq) -> Demux3/1, Sub2/2
  ChannelIn1/3 -> ChannelOut1/3
  ChannelIn1/2 -> ChannelOut1/2
  ChannelIn1/1 -> ChannelOut1/1
  dv/1 -> ChannelIn1/1
  dc/1 -> ChannelIn1/2
  valid_in/1 -> ChannelIn1/3
  axis_in/1 -> ChannelIn1/4
  ChannelOut1/1 -> qv/1
  ChannelOut1/2 -> qc/1
  ChannelOut1/3 -> valid_out/1
  ChannelOut1/4 -> axis_out/1
  Ready/1 -> ChannelOut1/22
  ChannelOut1/22 -> ready/1
  Mux4/1 -> SVM/2(ABin)
  I_Sat_Limit/1 -> ChannelIn1/14
  a2_f_cfg/1 -> ChannelIn1/16
  Torque/1 -> ChannelIn1/8
  Iw/1 -> ChannelIn1/7
  IntegralQ_in/1 -> ChannelIn1/9
  Iu/1 -> ChannelIn1/6
  b2_f_cfg/1 -> ChannelIn1/19
  b0_f_cfg/1 -> ChannelIn1/17
  phi_el/1 -> ChannelIn1/11
  IntegralD_in/1 -> ChannelIn1/10
  Kp/1 -> ChannelIn1/12
  Ki/1 -> ChannelIn1/13
  a1_f_cfg/1 -> ChannelIn1/15
  filt_disable_cfg/1 -> ChannelIn1/21
  d_y_k_2_f/1 -> ChannelIn1/25
  q_y_k_2_f1/1 -> ChannelIn1/29
  d_u_k_2_f/1 -> ChannelIn1/23
  q_u_k_2_f1/1 -> ChannelIn1/27
  q_y_k_1_f1/1 -> ChannelIn1/28
  d_y_k_1_f/1 -> ChannelIn1/24
  b1_f_cfg/1 -> ChannelIn1/18
  d_u_k_1_f/1 -> ChannelIn1/22
  xDCGain_f_cfg/1 -> ChannelIn1/20
  q_u_k_1_f1/1 -> ChannelIn1/26
  Convert11/1 -> [DCGain_f]
  Convert4/1 -> [a2_f]
  Convert10/1 -> [b2_f]
  Convert9/1 -> [b1_f]
  Mux1/1 -> [iuw]
  ChannelIn1/7 -> Mux1/2
  ChannelIn1/12 -> [kp]
  ChannelIn1/22 -> [d_u_k_1_f]
  ChannelIn1/26 -> [q_u_k_1_f]
  ChannelIn1/9 -> [int_q]
  ChannelIn1/14 -> [limit2]
  ChannelIn1/15 -> Convert1/1
  ChannelIn1/25 -> [d_y_k_2_f]
  Convert1/1 -> [a1_f]
  ChannelIn1/17 -> Convert8/1
  ChannelIn1/16 -> Convert4/1
  ChannelIn1/21 -> [filt_disable_cfg]
  ChannelIn1/18 -> Convert9/1
  ChannelIn1/24 -> [d_y_k_1_f]
  ChannelIn1/19 -> Convert10/1
  ChannelIn1/6 -> Mux1/1
  ChannelIn1/29 -> [q_y_k_2_f]
  ChannelIn1/28 -> [q_y_k_1_f]
  Convert8/1 -> [b0_f]
  ChannelIn1/10 -> [int_d]
  ChannelIn1/27 -> [q_u_k_2_f]
  ChannelIn1/11 -> [phi_el]
  ChannelIn1/23 -> [d_u_k_2_f]
  ChannelIn1/13 -> [ki]
  ChannelIn1/20 -> Convert11/1
  ChannelIn1/8 -> Mux2/2
  Max/1 -> ChannelIn1/5
  ChannelIn1/5 -> SVM/1(tmax)
  [Iq] -> ChannelOut1/20
  [IQ_out] -> Convert5/1
  [q_y_k_1_f] -> ChannelOut1/17
  [q_u_k_f] -> ChannelOut1/14
  Convert3/1 -> ChannelOut1/8
  [d_u_k_f] -> ChannelOut1/10
  [Vq_unfilt] -> ChannelOut1/18
  [Vd_unfilt] -> ChannelOut1/19
  [d_u_k_1_f] -> ChannelOut1/11
  Convert5/1 -> ChannelOut1/9
  [d_y_k_f] -> ChannelOut1/12
  [q_y_k_f] -> ChannelOut1/16
  [q_u_k_1_f] -> ChannelOut1/15
  [Id] -> ChannelOut1/21
  [d_y_k_1_f] -> ChannelOut1/13
  [ID_out] -> Convert3/1
  ChannelOut1/21 -> Id/1
  ChannelOut1/20 -> Iq/1
  ChannelOut1/10 -> dout_d_u_k_f/1
  ChannelOut1/18 -> Vq_unfilt/1
  ChannelOut1/14 -> dout_q_u_k_f/1
  ChannelOut1/12 -> dout_d_y_k_f/1
  ChannelOut1/13 -> dout_d_y_k_1_f/1
  ChannelOut1/15 -> dout_q_u_k_1_f/1
  ChannelOut1/8 -> IntegralD_out/1
  ChannelOut1/16 -> dout_q_y_k_f/1
  ChannelOut1/17 -> dout_q_y_k_1_f/1
  ChannelOut1/11 -> dout_d_u_k_1_f/1
  ChannelOut1/19 -> Vd_unfilt/1
  ChannelOut1/9 -> IntegralQ_out/1
  ChannelOut1/7 -> Vbeta/1
  ChannelOut1/6 -> Valpha/1
  SVM/1(Out_uvw) -> ChannelOut1/5
  ChannelOut1/5 -> uvw/1
  SVM/2(Out_sect) -> Terminator5/1

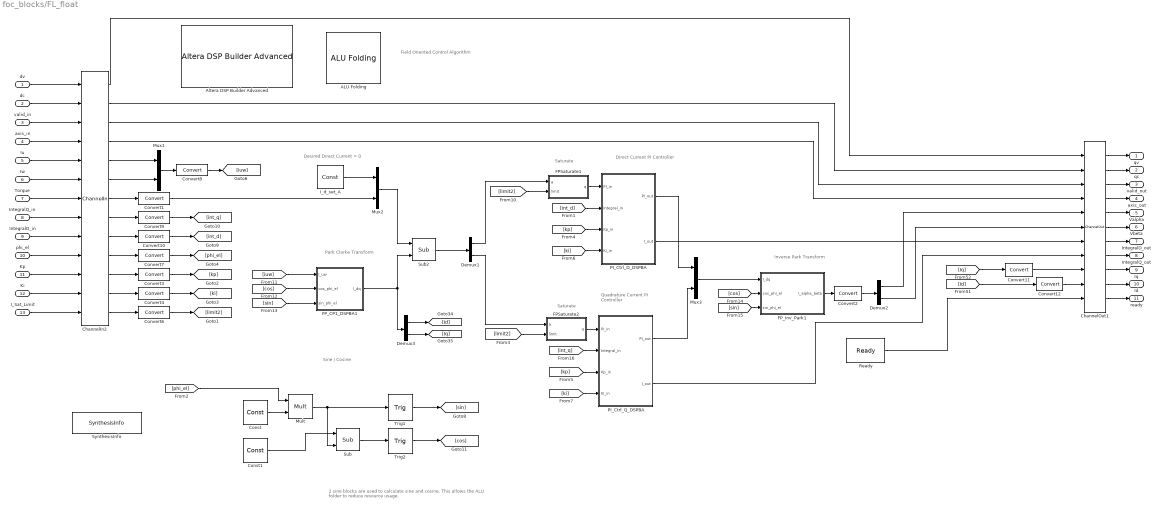
== system foc_blocks/FL_float ==
  note: Quadrature Current
      | PI Controller
  note: Direct Current
      | PI Controller
  note: Desired Direct Current = 0
  note: Inverse Park
      |  Transform
  note: Park Clarke
      |  Transform
  note: Saturate
  note: Saturate
  note: Sine / Cosine
  note: Field Oriented Control Algorithm
  note: 2 sine blocks are used to calculate sine and cosine.
      | This allows the ALU folder to reduce resource usage.
  dv : Inport
  dc : Inport  Port=2
  valid_in : Inport  Port=3
  axis_in : Inport  Port=4
  Iu : Inport  Port=5
  Iw : Inport  Port=6
  Torque : Inport  Port=7
  IntegralQ_in : Inport  Port=8
  IntegralD_in : Inport  Port=9
  phi_el : Inport  Port=10
  Kp : Inport  Port=11
  Ki : Inport  Port=12
  I_Sat_Limit : Inport  Port=13
  ALU Folding : DSPBAUtilities/ALU Folding  Description=Enables the new folder. When this block is placed in a subsystem, all primitive subsystems at the level it is placed and below will be passed to the folder. DSP Builder will then generate folded subsystems which can be placed back into the existing design.  version=20130913  genModelFileName=folded_model.xml  sampleRate=SampleRate  numChannels=1  maxLatency=LatencyConstraint  inputFormat=Parallel  outputFormat=Parallel  latchOutputs=off  originalRate=off  hasIdleState=off  padInputs=off  simRate=Data rate
  Altera DSP Builder Advanced : AlteraGenericMotorLibrary/FP_Cur_Ctrl_DSPBA/Altera DSP Builder Advanced  SystemSampleTime=-1  VariantActivationTime=update diagram  Latency=0  AutoFrameSizeCalculation=off
  ChannelIn2 : DSPBAPrim/ChannelIn  primtype=channelin  nInputs=dspba_internal_get_channel_ports(gcb)  nOutputs=dspba_internal_get_channel_ports(gcb)  omode=Inherit via internal rule  otype=sfix(16)  scale=2^-15  rndmethod=Unbiased  factor=1  satmethod=Symmetric  shift_vec=[0 1 2 -1]  value=11  inPortNames=['v'; 'c'; '0'; '1'; '2'; '3'; '4'; '5'; '6'; '7'; '8'; '9'; 'A'; 'B'; 'D'; 'E'; 'F'; 'G'; 'H'; 'I'; 'J'; 'K'; 'L'; 'M'; 'N'; 'O'; 'P'; 'Q'; 'R'; 'S'; 'T'; 'U'; 'W'; 'X'; 'Y'; 'Z']  outPortNames=['v'; 'c'; '0'; '1'; '2'; '3'; '4'; '5'; '6'; '7'; '8'; '9'; 'A'; 'B'; 'D'; 'E'; 'F'; 'G'; 'H'; 'I'; 'J'; 'K'; 'L'; 'M'; 'N'; 'O'; 'P'; 'Q'; 'R'; 'S'; 'T'; 'U'; 'W'; 'X'; 'Y'; 'Z']  dspbaimage=dspba_prim.jpg  text=fprintf('In');  style=Optimised  dataSignals=11  foldingEnabled=off  channels=1  sampleRate=200  packetBeginPresent=off  packetBeginEnabled=off  visibilities=dspba_ChannelInVis(gcb)  latencyCorrection=0  scheduleOrigin=off  version=20141013
  ChannelOut1 : DSPBAPrim/ChannelOut  primtype=channelout  nInputs=dspba_internal_get_channel_ports(gcb)  nOutputs=dspba_internal_get_channel_ports(gcb)  omode=Inherit via internal rule  otype=sfix(16)  scale=2^-15  rndmethod=Unbiased  factor=1  satmethod=Symmetric  shift_vec=[0 1 2 -1]  value=9  inPortNames=['v'; 'c'; '0'; '1'; '2'; '3'; '4'; '5'; '6'; '7'; '8'; '9'; 'A'; 'B'; 'D'; 'E'; 'F'; 'G'; 'H'; 'I'; 'J'; 'K'; 'L'; 'M'; 'N'; 'O'; 'P'; 'Q'; 'R'; 'S'; 'T'; 'U'; 'W'; 'X'; 'Y'; 'Z']  outPortNames=['v'; 'c'; '0'; '1'; '2'; '3'; '4'; '5'; '6'; '7'; '8'; '9'; 'A'; 'B'; 'D'; 'E'; 'F'; 'G'; 'H'; 'I'; 'J'; 'K'; 'L'; 'M'; 'N'; 'O'; 'P'; 'Q'; 'R'; 'S'; 'T'; 'U'; 'W'; 'X'; 'Y'; 'Z']  dspbaimage=dspba_prim.jpg  text=fprintf('Out%s', AdvDSPBChannelOutDisplay(latency));  style=Optimised  dataSignals=9  foldingEnabled=off  channels=1  sampleRate=200  packetBeginPresent=off  packetBeginEnabled=off  visibilities=dspba_ChannelOutVis(gcb)  latency=159  latencyCorrection=0  version=20141013
  Const : DSPBAPrim/Const  primtype=const  nInputs=0  nOutputs=1  omode=Specify via dialog  otype=fpDT  scale=1  rndmethod=Unbiased  factor=1  satmethod=Symmetric  shift_vec=[0 1 2 -1]  value=2  inPortNames=['+'; '+';]  outPortNames=[' ']  dspbaimage=dspba_prim.jpg  text=fprintf('%s', num2str(value));  style=Optimised  visibilities=8 + 1024  floatPrecision=float26_m17  version=20120820
  Const1 : DSPBAPrim/Const  primtype=const  nInputs=0  nOutputs=1  omode=Specify via dialog  otype=fpDT  scale=1  rndmethod=Unbiased  factor=1  satmethod=Symmetric  shift_vec=[0 1 2 -1]  value=1/2  inPortNames=['+'; '+';]  outPortNames=[' ']  dspbaimage=dspba_prim.jpg  text=fprintf('%s', num2str(value));  style=Optimised  visibilities=8 + 1024  floatPrecision=float26_m17  version=20120820
  Convert{1,3..4,6..10} (8 alike) : DSPBAPrim/Convert  primtype=convert  nInputs=1  nOutputs=1  omode=Specify via dialog  otype=fpDT  scale=1  rndmethod=Unbiased  factor=1  satmethod=None  shift_vec=[0 1 2 -1]  value=round([0:255]/17)  inPortNames=[' '; ' ';]  outPortNames=[' '; 'c']  dspbaimage=dspba_prim.jpg  text=fprintf('convert');  style=Optimised  visibilities=8+64+256  clipdetect=off  floatPrecision=float32_m23  advOptions=[]  version=20130211
  Convert11 : DSPBAPrim/Convert  primtype=convert  nInputs=1  nOutputs=1  omode=Specify via dialog  otype=constOType  scale=constScale  rndmethod=Truncate  factor=1  satmethod=None  shift_vec=[0 1 2 -1]  value=round([0:255]/17)  inPortNames=[' '; ' ';]  outPortNames=[' '; 'c']  dspbaimage=dspba_prim.jpg  text=fprintf('convert');  style=Optimised  visibilities=8+64+256  clipdetect=off  floatPrecision=float32_m23  advOptions=[]  version=20130211
  Convert12 : DSPBAPrim/Convert  primtype=convert  nInputs=1  nOutputs=1  omode=Specify via dialog  otype=constOType  scale=constScale  rndmethod=Truncate  factor=1  satmethod=None  shift_vec=[0 1 2 -1]  value=round([0:255]/17)  inPortNames=[' '; ' ';]  outPortNames=[' '; 'c']  dspbaimage=dspba_prim.jpg  text=fprintf('convert');  style=Optimised  visibilities=8+64+256  clipdetect=off  floatPrecision=float32_m23  advOptions=[]  version=20130211
  Convert2 : DSPBAPrim/Convert  primtype=convert  nInputs=1  nOutputs=1  omode=Specify via dialog  otype=constOType  scale=constScale  rndmethod=Truncate  factor=1  satmethod=None  shift_vec=[0 1 2 -1]  value=round([0:255]/17)  inPortNames=[' '; ' ';]  outPortNames=[' '; 'c']  dspbaimage=dspba_prim.jpg  text=fprintf('convert');  style=Optimised  visibilities=8+64+256  clipdetect=off  floatPrecision=float32_m23  advOptions=[]  version=20130211
  Demux1 : Demux  Outputs=2
  Demux2 : Demux  Outputs=2
  Demux3 : Demux  Outputs=2
  FPSaturate1 : Subsystem
      mask Display: color('w');fprintf('FP Var Sat\n');port_label('input',1,'a');port_label('input',2,'limit');port_label('output',1,'q');
  FPSaturate2 : Subsystem
      mask Display: color('w');fprintf('FP Var Sat\n');port_label('input',1,'a');port_label('input',2,'limit');port_label('output',1,'q');
  FP_CP1_DSPBA1 : Subsystem  Description=Clarke & Park Transforms
  FP_Inv_Park1 : Subsystem  Description=Inverse Park & Clarke transforms
  I_d_set_A : DSPBAPrim/Const  primtype=const  nInputs=0  nOutputs=1  omode=Specify via dialog  otype=fpDT  scale=1  rndmethod=Unbiased  factor=1  satmethod=Symmetric  shift_vec=[0 1 2 -1]  value=0  inPortNames=['+'; '+';]  outPortNames=[' ']  dspbaimage=dspba_prim.jpg  text=fprintf('%s', num2str(value));  style=Optimised  visibilities=8 + 1024  floatPrecision=float32_m23  version=20120820
  Mult : DSPBAPrim/Mult  primtype=mult  nInputs=2  nOutputs=1  omode=Inherit via internal rule  otype=sfix(16)  scale=2^-15  rndmethod=Unbiased  factor=1  satmethod=Symmetric  shift_vec=[0 1 2 -1]  value=0  inPortNames=[' '; ' ';]  outPortNames=[' ']  dspbaimage=dspba_prim.jpg  text=fprintf('X');  style=Optimised  visibilities=8+2^18+2^19  floatPrecision=float32_m23  floatRounding=faithful  advOptions=[]  version=20130115
  Mux1 : Mux  Inputs=2
  Mux2 : Mux  Inputs=2
  Mux3 : Mux  Inputs=2
  PI_Ctrl_D_DSPBA : Subsystem
  PI_Ctrl_Q_DSPBA : Subsystem
  Ready : DSPBAPrim/Ready  primtype=ready  nInputs=0  nOutputs=1  omode=Inherit via internal rule  otype=ufix(1)  scale=2^-0  rndmethod=Unbiased  factor=1  satmethod=Asymmetric  shift_vec=[]  value=1  inPortNames=['']  outPortNames=[' ']  dspbaimage=dspba_prim.jpg  text=fprintf('Ready');  style=Processor  visibilities=0  floatPrecision=float32_m23  version=20131024
  Sub : DSPBAPrim/Sub  primtype=sub  nInputs=2  nOutputs=1  omode=Inherit via internal rule with word growth  otype=sfix(16)  scale=2^-15  rndmethod=Unbiased  factor=1  satmethod=Symmetric  shift_vec=[0 1 2 -1]  value=0  inPortNames=['+'; '-';]  outPortNames=[' ']  dspbaimage=dspba_prim.jpg  text=fprintf('-');  style=Optimised  visibilities=8+2^17+2^18  floatRounding=faithful  advOptions=[]  version=20130115
  Sub2 : DSPBAPrim/Sub  primtype=sub  nInputs=2  nOutputs=1  omode=Inherit via internal rule with word growth  otype=sfix(16)  scale=2^-15  rndmethod=Unbiased  factor=1  satmethod=Symmetric  shift_vec=[0 1 2 -1]  value=0  inPortNames=['+'; '-';]  outPortNames=[' ']  dspbaimage=dspba_prim.jpg  text=fprintf('-');  style=Optimised  visibilities=8  floatRounding=faithful  advOptions=[]  version=20130115
  SynthesisInfo : DSPBAPrim/SynthesisInfo  primtype=synthinfo  nInputs=0  nOutputs=0  omode=Inherit via internal rule  otype=sfix(16)  scale=2^-15  rndmethod=Truncate  factor=1  satmethod=Symmetric  shift_vec=[0 1 2 -1]  value=99  inPortNames=[' '; ' ';]  outPortNames=[' ']  dspbaimage=dspba_prim_ctrl.jpg  text=fprintf('Style=%s', style);  style=Scheduled  visibilities=32768  constraintInUse=off  constraintRelation=>  constraintLimit=2  bitAccurate=off  version=20150220
  Trig1 : DSPBAPrim/Trig  primtype=trigfunc  nInputs=1  nOutputs=1  omode=Inherit via internal rule  otype=sfix(16)  scale=2^-15  rndmethod=Unbiased  factor=1  satmethod=Symmetric  shift_vec=[0 1 2 -1]  value=round([0:255]/17)  inPortNames=[' '; ' ';]  outPortNames=[' ']  dspbaimage=dspba_prim_float.jpg  text=fprintf('sin(a)');  style=Optimised  visibilities=2^17+2^18  functionExpr=sin(pi*x)  advOptions=[]  version=20140803
  Trig2 : DSPBAPrim/Trig  primtype=trigfunc  nInputs=1  nOutputs=1  omode=Inherit via internal rule  otype=sfix(16)  scale=2^-15  rndmethod=Unbiased  factor=1  satmethod=Symmetric  shift_vec=[0 1 2 -1]  value=round([0:255]/17)  inPortNames=[' '; ' ';]  outPortNames=[' ']  dspbaimage=dspba_prim_float.jpg  text=fprintf('sin(a)');  style=Optimised  visibilities=2^17+2^18  functionExpr=sin(pi*x)  advOptions=[]  version=20140803
  qv : Outport
  qc : Outport  Port=2
  valid_out : Outport  Port=3
  axis_out : Outport  Port=4
  Valpha : Outport  Port=5
  Vbeta : Outport  Port=6
  IntegralD_out : Outport  Port=7
  IntegralQ_out : Outport  Port=8
  Iq : Outport  Port=9
  Id : Outport  Port=10
  ready : Outport  Port=11
  wires:
  Convert7/1 -> [phi_el]
  Convert10/1 -> [int_d]
  Convert9/1 -> [int_q]
  Trig2/1 -> [cos]
  Trig1/1 -> [sin]
  Sub/1 -> Trig2/1
  Mult/1 -> Sub/2, Trig1/1
  Const1/1 -> Sub/1
  Const/1 -> Mult/2
  [phi_el] -> Mult/1
  ChannelIn2/1 -> ChannelOut1/1
  ChannelIn2/2 -> ChannelOut1/2
  ChannelIn2/5 -> Mux1/1
  ChannelIn2/6 -> Mux1/2
  ChannelIn2/3 -> ChannelOut1/3
  FPSaturate2/1(q) -> PI_Ctrl_Q_DSPBA/1(PI_in)
  FPSaturate1/1(q) -> PI_Ctrl_D_DSPBA/1(PI_in)
  PI_Ctrl_Q_DSPBA/2(I_out) -> ChannelOut1/8
  PI_Ctrl_D_DSPBA/2(I_out) -> ChannelOut1/7
  PI_Ctrl_D_DSPBA/1(PI_out) -> Mux3/1
  PI_Ctrl_Q_DSPBA/1(PI_out) -> Mux3/2
  Mux3/1 -> FP_Inv_Park1/1(I_dq)
  FP_Inv_Park1/1(I_alpha_beta) -> Convert2/1
  Demux2/1 -> ChannelOut1/5
  Demux2/2 -> ChannelOut1/6
  dv/1 -> ChannelIn2/1
  valid_in/1 -> ChannelIn2/3
  dc/1 -> ChannelIn2/2
  Iu/1 -> ChannelIn2/5
  Iw/1 -> ChannelIn2/6
  Torque/1 -> ChannelIn2/7
  I_d_set_A/1 -> Mux2/1
  Mux2/1 -> Sub2/1
  Sub2/1 -> Demux1/1
  Demux1/1 -> FPSaturate1/1(a)
  Demux1/2 -> FPSaturate2/1(a)
  [int_q] -> PI_Ctrl_Q_DSPBA/2(Integral_in)
  [kp] -> PI_Ctrl_Q_DSPBA/3(Kp_in)
  [ki] -> PI_Ctrl_Q_DSPBA/4(Ki_in)
  [limit2] -> FPSaturate2/2(limit)
  [int_d] -> PI_Ctrl_D_DSPBA/2(Integral_in)
  [kp] -> PI_Ctrl_D_DSPBA/3(Kp_in)
  [ki] -> PI_Ctrl_D_DSPBA/4(Ki_in)
  [limit2] -> FPSaturate1/2(limit)
  [iuw] -> FP_CP1_DSPBA1/1(I_uw)
  [cos] -> FP_CP1_DSPBA1/2(cos_phi_el)
  [sin] -> FP_CP1_DSPBA1/3(sin_phi_el)
  Mux1/1 -> Convert8/1
  [cos] -> FP_Inv_Park1/2(cos_phi_el)
  [sin] -> FP_Inv_Park1/3(sin_phi_el)
  Convert6/1 -> [limit2]
  Convert4/1 -> [ki]
  Convert3/1 -> [kp]
  Convert8/1 -> [iuw]
  Convert1/1 -> Mux2/2
  axis_in/1 -> ChannelIn2/4
  ChannelIn2/4 -> ChannelOut1/4
  Convert2/1 -> Demux2/1
  Ready/1 -> ChannelOut1/11
  IntegralQ_in/1 -> ChannelIn2/8
  IntegralD_in/1 -> ChannelIn2/9
  phi_el/1 -> ChannelIn2/10
  Kp/1 -> ChannelIn2/11
  Ki/1 -> ChannelIn2/12
  ChannelIn2/7 -> Convert1/1
  ChannelIn2/8 -> Convert9/1
  ChannelIn2/9 -> Convert10/1
  ChannelIn2/10 -> Convert7/1
  ChannelIn2/11 -> Convert3/1
  ChannelIn2/12 -> Convert4/1
  ChannelOut1/1 -> qv/1
  ChannelOut1/2 -> qc/1
  ChannelOut1/3 -> valid_out/1
  ChannelOut1/4 -> axis_out/1
  ChannelOut1/5 -> Valpha/1
  ChannelOut1/6 -> Vbeta/1
  ChannelOut1/7 -> IntegralD_out/1
  ChannelOut1/8 -> IntegralQ_out/1
  ChannelOut1/11 -> ready/1
  FP_CP1_DSPBA1/1(I_dq) -> Demux3/1, Sub2/2
  Demux3/1 -> [Id]
  Demux3/2 -> [Iq]
  [Iq] -> Convert11/1
  [Id] -> Convert12/1
  ChannelOut1/9 -> Iq/1
  ChannelOut1/10 -> Id/1
  Convert11/1 -> ChannelOut1/9
  Convert12/1 -> ChannelOut1/10
  ChannelIn2/13 -> Convert6/1
  I_Sat_Limit/1 -> ChannelIn2/13
